simulink model "force_control"  (R2023a)
settings: Solver=VariableStepAuto  StartTime=0.0  StopTime=10.0  RelTol=1e-3
undefined symbols (not defined in the file): dqi, fd, K, KD, KF, KI, KP, Md, Md_inv, qi, robot, xr
settings Model: Creator=franc  LastModifiedBy=franc

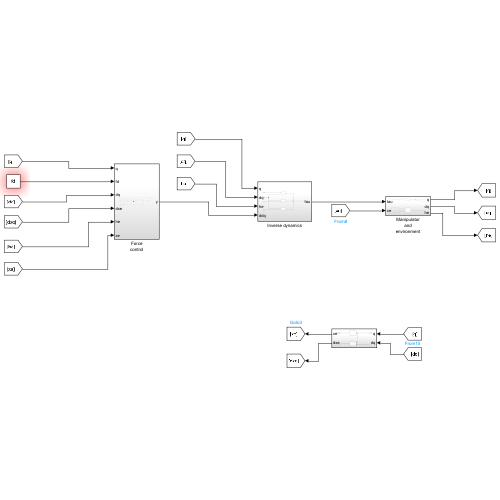
[thumbnail: Simulink's stored preview of the top-level diagram]
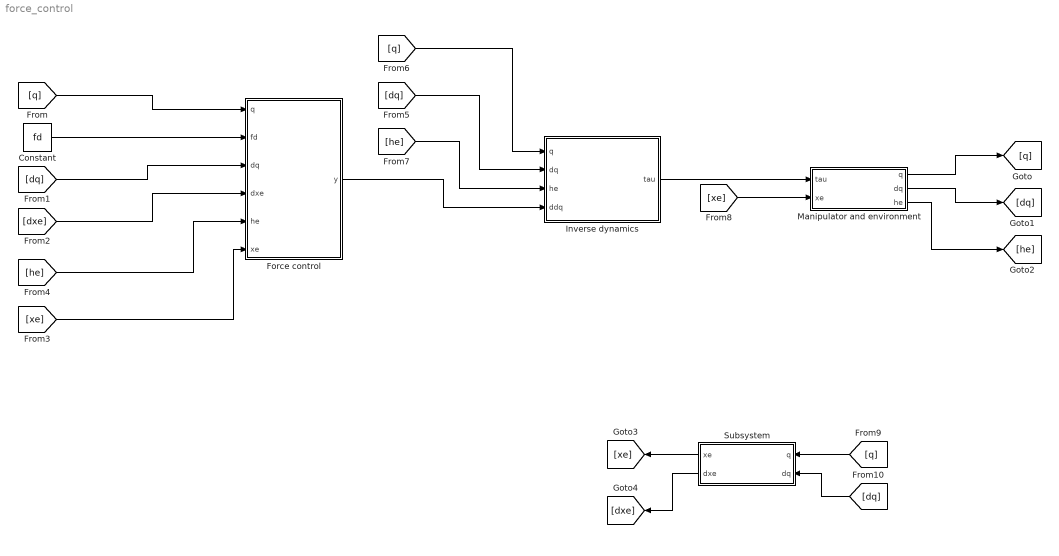
== system force_control ==
  Constant : Constant  Value=fd
  Force control : Subsystem
  Inverse dynamics : Subsystem
  Manipulator and environment : Subsystem
  Subsystem : Subsystem
  wires:
  Constant/1 -> Force control/2(fd)
  [q] -> Force control/1(q)
  [dq] -> Force control/3(dq)
  [xe] -> Force control/6(xe)
  [dxe] -> Force control/4(dxe)
  [he] -> Force control/5(he)
  Force control/1(y) -> Inverse dynamics/4(ddq)
  [dq] -> Inverse dynamics/2(dq)
  [q] -> Inverse dynamics/1(q)
  [he] -> Inverse dynamics/3(he)
  Inverse dynamics/1(tau) -> Manipulator and environment/1(tau)
  [xe] -> Manipulator and environment/2(xe)
  Manipulator and environment/1(q) -> [q]
  Manipulator and environment/2(dq) -> [dq]
  Manipulator and environment/3(he) -> [he]
  Subsystem/1(xe) -> [xe]
  Subsystem/2(dxe) -> [dxe]
  [q] -> Subsystem/1(q)
  [dq] -> Subsystem/2(dq)

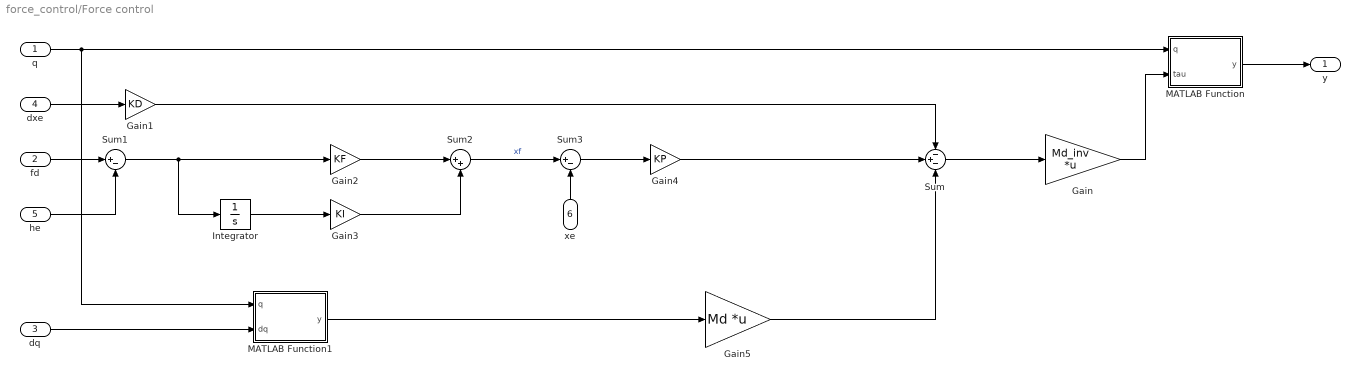
== system force_control/Force control ==
  q : Inport
  fd : Inport  Port=2
  dq : Inport  Port=3
  dxe : Inport  Port=4
  he : Inport  Port=5
  xe : Inport  Port=6
  Gain : Gain  Gain=Md_inv  Multiplication=Matrix(K*u)
  Gain1 : Gain  Gain=KD
  Gain2 : Gain  Gain=KF
  Gain3 : Gain  Gain=KI
  Gain4 : Gain  Gain=KP
  Gain5 : Gain  Gain=Md  Multiplication=Matrix(K*u)
  Integrator : Integrator
  MATLAB Function : MATLAB Function  TreatAsAtomicUnit=on
  MATLAB Function1 : MATLAB Function  TreatAsAtomicUnit=on
  Sum : Sum  Inputs=-+-
  Sum1 : Sum  Inputs=|+-
  Sum2 : Sum  Inputs=|++
  Sum3 : Sum  Inputs=|+-
  y : Outport
  wires:
  MATLAB Function/1(y) -> y/1
  q/1 -> MATLAB Function/1(q), MATLAB Function1/1(q)
  Gain/1 -> MATLAB Function/2(tau)
  Sum/1 -> Gain/1
  dxe/1 -> Gain1/1
  Gain1/1 -> Sum/1
  fd/1 -> Sum1/1
  he/1 -> Sum1/2
  Sum1/1 -> Integrator/1, Gain2/1
  Integrator/1 -> Gain3/1
  Gain2/1 -> Sum2/1
  Gain3/1 -> Sum2/2
  Sum2/1 -> Sum3/1  "xf"
  xe/1 -> Sum3/2
  Gain4/1 -> Sum/2
  Sum3/1 -> Gain4/1
  dq/1 -> MATLAB Function1/2(dq)
  Gain5/1 -> Sum/3
  MATLAB Function1/1(y) -> Gain5/1

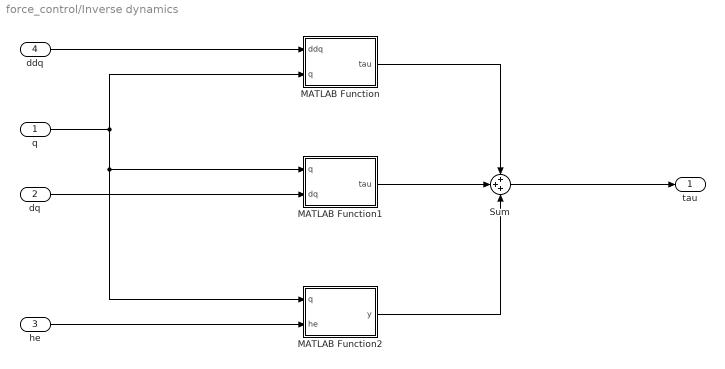
== system force_control/Inverse dynamics ==
  q : Inport
  dq : Inport  Port=2
  he : Inport  Port=3
  ddq : Inport  Port=4
  MATLAB Function : MATLAB Function  TreatAsAtomicUnit=on
  MATLAB Function1 : MATLAB Function  TreatAsAtomicUnit=on
  MATLAB Function2 : MATLAB Function  TreatAsAtomicUnit=on
  Sum : Sum  Inputs=+++
  tau : Outport
  wires:
  he/1 -> MATLAB Function2/2(he)
  dq/1 -> MATLAB Function1/2(dq)
  q/1 -> MATLAB Function2/1(q), MATLAB Function1/1(q), MATLAB Function/2(q)
  ddq/1 -> MATLAB Function/1(ddq)
  MATLAB Function1/1(tau) -> Sum/2
  MATLAB Function/1(tau) -> Sum/1
  MATLAB Function2/1(y) -> Sum/3
  Sum/1 -> tau/1

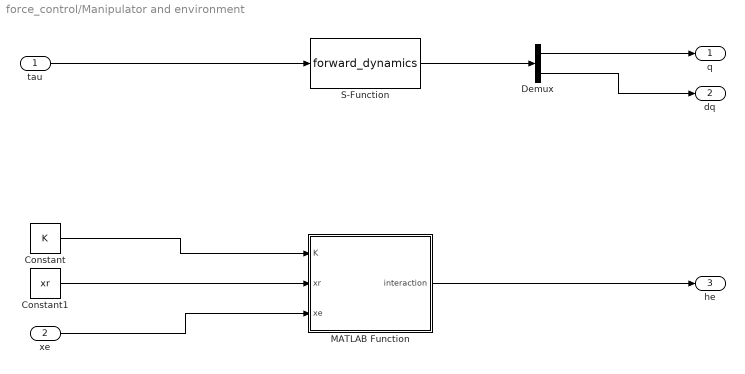
== system force_control/Manipulator and environment ==
  tau : Inport
  xe : Inport  Port=2
  Constant : Constant  Value=K
  Constant1 : Constant  Value=xr
  Demux : Demux  Outputs=2
  MATLAB Function : MATLAB Function  TreatAsAtomicUnit=on
  S-Function : S-Function  FunctionName=forward_dynamics  Parameters=robot,qi,dqi  SFunctionDeploymentMode=off  EnableBusSupport=off
  q : Outport
  dq : Outport  Port=2
  he : Outport  Port=3
  wires:
  tau/1 -> S-Function/1
  S-Function/1 -> Demux/1
  Demux/1 -> q/1
  Demux/2 -> dq/1
  Constant/1 -> MATLAB Function/1(K)
  Constant1/1 -> MATLAB Function/2(xr)
  xe/1 -> MATLAB Function/3(xe)
  MATLAB Function/1(interaction) -> he/1

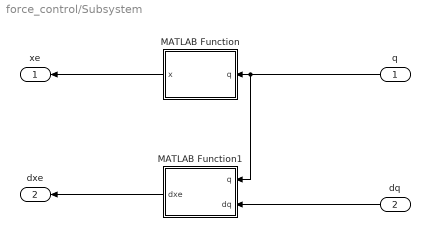
== system force_control/Subsystem ==
  q : Inport
  dq : Inport  Port=2
  MATLAB Function : MATLAB Function  TreatAsAtomicUnit=on
  MATLAB Function1 : MATLAB Function  TreatAsAtomicUnit=on
  xe : Outport
  dxe : Outport  Port=2
  wires:
  q/1 -> MATLAB Function1/1(q), MATLAB Function/1(q)
  MATLAB Function/1(x) -> xe/1
  dq/1 -> MATLAB Function1/2(dq)
  MATLAB Function1/1(dxe) -> dxe/1

== matlab function force_control/Force control/MATLAB Function ==
  data: q input; y output; tau input
function y = Ja_inv(q,tau)

y = get_Ja_inverse_as_9(q(1),q(2),q(3))* tau;

== matlab function force_control/Inverse dynamics/MATLAB Function ==
  data: ddq input; q input; tau output
function tau = B(ddq,q)

tau = get_B_as_7(q(1),q(3)) * ddq;

== matlab function force_control/Inverse dynamics/MATLAB Function1 ==
  data: q input; tau output; dq input
function tau = n(q,dq)

tau = get_n_as_7(q(1),q(3),dq(1),dq(3));

== matlab function force_control/Inverse dynamics/MATLAB Function2 ==
  data: q input; y output; he input
function y = J(q,he)

y = get_Ja_as_9(q(1),q(2),q(3))'*he;

== matlab function force_control/Manipulator and environment/MATLAB Function ==
  data: K input; interaction output; xr input; xe input
function interaction = hde(K,xr,xe)

if xe(3) < xr(3)
    interaction = K * (xe-xr);
else
    interaction = zeros(6,1);
end

== matlab function force_control/Subsystem/MATLAB Function ==
  data: q input; x output
function x = K(q)

x = get_k_as_9(q(1),q(2),q(3));

== matlab function force_control/Subsystem/MATLAB Function1 ==
  data: q input; dxe output; dq input
function dxe = Ja(q,dq)

dxe = get_Ja_as_9(q(1),q(2),q(3))*dq;

== matlab function force_control/Force control/MATLAB Function1 ==
  data: q input; y output; dq input
function y = dJa(q,dq)

y = get_derivative_Ja_as_9(q(1),q(2),q(3),dq(1),dq(2),dq(3))*dq;
